simulink model "Thesis_model"  (R2023b)
settings: Solver=FixedStepAuto  StartTime=0  StopTime=24*3600*3  FixedStep=3600  RelTol=1e-3
undefined symbols (not defined in the file): C_Battery_kWh, Davies, demand, Hay, Max_charge_potential, P_Inv_W_max, path_carnot, phase, plugin_out, PV_W, req_charge, req_SOC
libraries: carnot x13, rllib x1
settings Model: Creator=Rohan  LastModifiedBy=Rohan
settings SolverCC: EnableFixedStepZeroCrossing=on

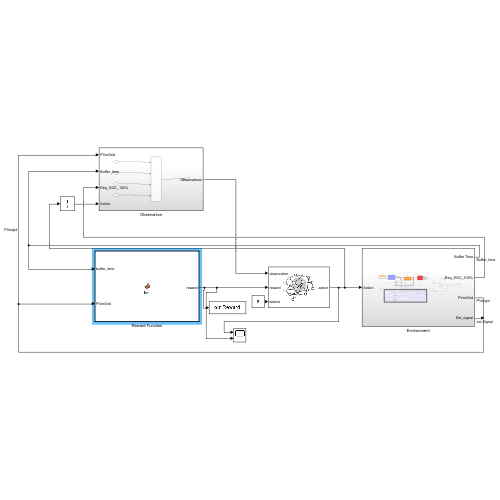
[thumbnail: Simulink's stored preview of the top-level diagram]
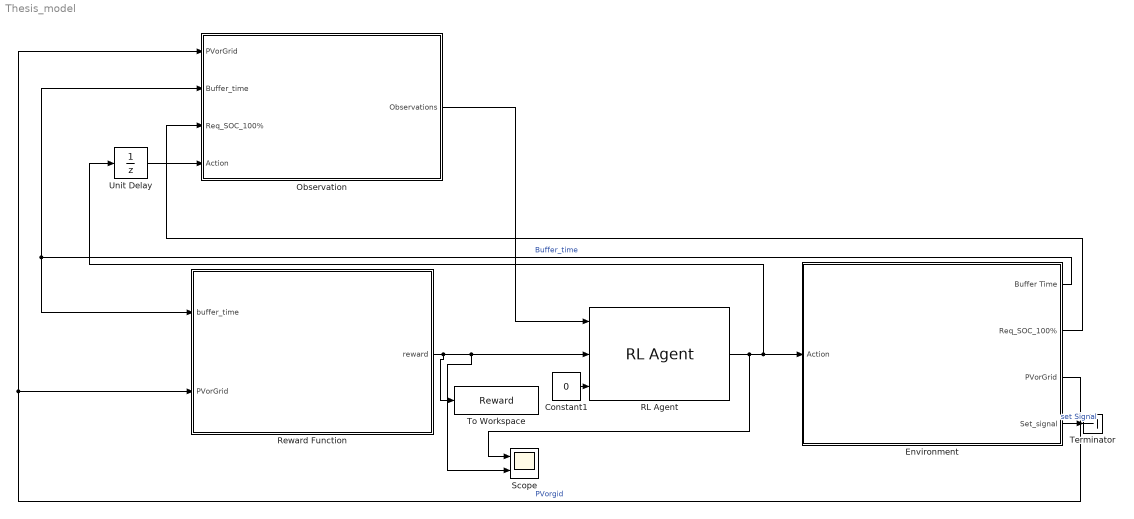
== system Thesis_model ==
  Constant1 : Constant  Value=0
  Environment : Subsystem
  Observation : Subsystem
  RL Agent : rllib/RL Agent  Agent=agentDQN_Trained  ExternalActionAsInput=off  ProvideLastAction=off  ProvideCumRwd=off  TreatAsDirectFeedthrough=on  UseStrictObservationDataTypes=off
  Reward Function : MATLAB Function  TreatAsAtomicUnit=on
  Scope : Scope  NumInputPorts=2
  Terminator : Terminator
  To Workspace : ToWorkspace  VariableName=Reward  SampleTime=-1
  Unit Delay : UnitDelay  SampleTime=-1  HasFrameUpgradeWarning=on
  wires:
  Reward Function/1(reward) -> To Workspace/1, Scope/2, RL Agent/2
  Environment/1(Buffer Time) -> Observation/2(Buffer_time), Reward Function/1(buffer_time)  "Buffer_time"
  Observation/1(Observations) -> RL Agent/1
  Constant1/1 -> RL Agent/3
  Environment/2(Req_SOC_100%) -> Observation/3(Req_SOC_100%)
  Environment/3(PVorGrid) -> Observation/1(PVorGrid), Reward Function/2(PVorGrid)  "PVorgid"
  RL Agent/1 -> Scope/1, Environment/1(Action), Unit Delay/1
  Unit Delay/1 -> Observation/4(Action)
  Environment/4(Set_signal) -> Terminator/1  "set Signal"

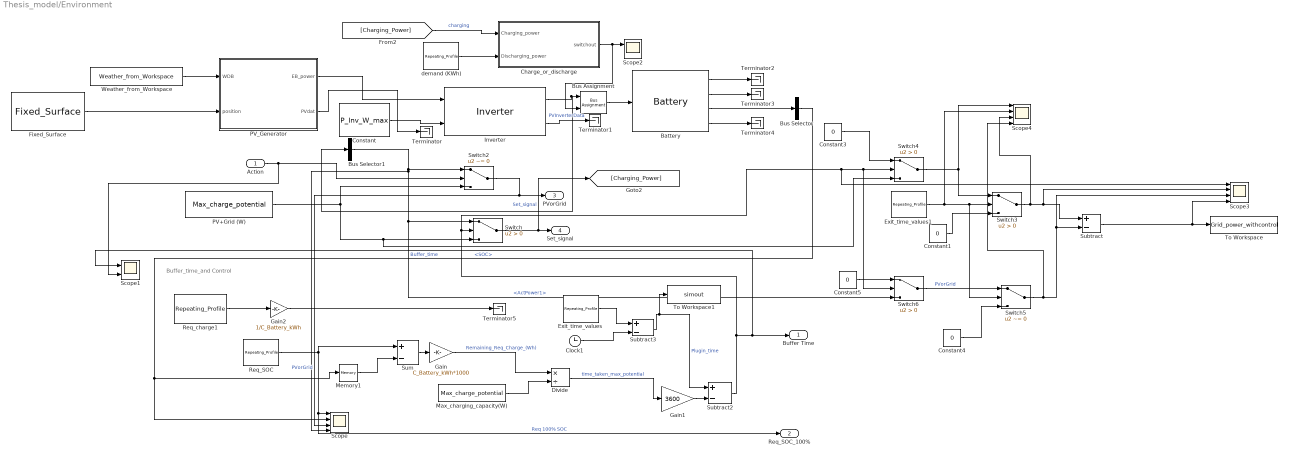
== system Thesis_model/Environment ==
  note: Buffer_time_and Control
  Action : Inport
  Battery : carnot/Storage/Electric/Battery  cap_kWh=C_Battery_kWh  eta_ch=1  eta_dis=1  cap0=Initial_SOC  SOC_max=1  SOC_min=0  Pmax=10000  Pmin=-10000  P_standby=0
      settings: SourceProductName=Carnot
  Bus Assignment : BusAssignment  AssignedSignals=ActPower1
  Bus Selector : BusSelector  OutputSignals=SOC
  Bus Selector1 : BusSelector  OutputSignals=ActPower1
  Charge_or_discharge : Subsystem
  Clock1 : Clock
  Constant : Constant  Value=P_Inv_W_max
  Constant{1,3..5} (4 alike) : Constant  Value=0
  Divide : Product  Inputs=*/
  Exit_time_values : carnot/Load/General/Repeating_Profile  period=plugin_out(end,1)  rep_seq_t=plugin_out(:,1)'  rep_seq_d=[1 ]*3600  rep_seq_y=plugin_out(:,2)'
      settings: SourceProductName=Carnot
  Exit_time_values1 : carnot/Load/General/Repeating_Profile  period=plugin_out(end,1)  rep_seq_t=plugin_out(:,1)'  rep_seq_d=[1 ]*3600  rep_seq_y=plugin_out(:,2)'
      settings: SourceProductName=Carnot
  Fixed_Surface : carnot/Weather/Fixed_Surface  colangle=30  colazi=0  colrot=0
      settings: SourceProductName=Carnot
  Gain : Gain  Gain=C_Battery_kWh*1000
  Gain1 : Gain  Gain=3600
  Gain2 : Gain  Gain=1/C_Battery_kWh
  Inverter : carnot/Source/Electric_Generator/Inverter  PathName=fullfile(path_carnot('libsl'), 'Source','Electric_Generator','Inverter','parameter_set')  FileName='<user defined>'  userPath=off  userParam=on  Pacnom=P_Inv_W  nphase=1-phase  U=230  f=50  PstepsEta=[0 0.1 0.2 0.25 0.3 0.5 0.75 1]  Eta=[0 0.948 0.966 0.969 0.97 0.972 0.97 0.967]  P_standby=0
      settings: SourceProductName=Carnot
  Max_charging_capacity(W) : Constant  Value=Max_charge_potential
  Memory1 : Memory
  PV+Grid (W) : Constant  Value=Max_charge_potential
  PV_Generator : Subsystem  AncestorBlock=carnot/Source/Electric_Generator/PV_Generator  mask(PV_Module_simple){Wp=PV_W, delta_Wp_K=0.0047, fgen=0.91 % 0.06 power missmatch, 0.01 diodes, 0.02 data sheet tolerance}
      mask prompts: Wp "Peak power of the generator [W]"; delta_Wp_K "Temperature coefficient Pmax 1/K"; fgen "efficiency generator field (lossses in diodes, power missmatch, dirt)"
      mask help:
      | This block simultes a PV module or generatater and calculates the DC power based on the parameters:
      | - Wp of one module or generator at STC [W]
      | - temperature coefficient of Pmax [1/K]
      | - dirt and degradation effects
      | The output DC power of the PV generator is ActPower1 in EB (power only)
      mask Help: web(fullfile(path_carnot('help'),'PV_Generator.html'),'-helpbrowser')
      mask Display: plot(0,0,100,100,[10,40,90,60,10],[10,90,90,10,10],[37,53,60,43,37],[70,70,86,86,70],[60,75,82,67,60],[70,71,86,86,70],[35,30,43,51,35],[65,50,49,65,65],[51,67,73,58,51],[50,50,66,66,50],[28,20,36,43,28],[41,23,23,41,41],[49,44,58,65,49],[41,23,22,41,41])
  Req_SOC : carnot/Load/General/Repeating_Profile  period=req_SOC(end,1)  rep_seq_t=req_SOC(:,1)'  rep_seq_d=[1 ]*3600  rep_seq_y=req_SOC(:,2)'
      settings: SourceProductName=Carnot
  Req_charge1 : carnot/Load/General/Repeating_Profile  period=req_charge(end,1)  rep_seq_t=req_charge(:,1)'  rep_seq_d=3600  rep_seq_y=req_charge(:,2)'
      settings: SourceProductName=Carnot
  Scope : Scope  NumInputPorts=4
  Scope1 : Scope  NumInputPorts=2
  Scope2 : Scope  NumInputPorts=2
  Scope3 : Scope  NumInputPorts=4
  Scope4 : Scope  NumInputPorts=4
  Subtract : Sum  Inputs=+-
  Subtract2 : Sum  Inputs=+-
  Subtract3 : Sum  Inputs=+-
  Sum : Sum  Inputs=|+-
  Switch : Switch  Criteria=u2 > Threshold  RndMeth=Zero  SaturateOnIntegerOverflow=off  InputSameDT=off
  Switch2 : Switch  Criteria=u2 ~= 0  Threshold=0.5  ZeroCross=off  SaturateOnIntegerOverflow=off  InputSameDT=off
  Switch3 : Switch  Criteria=u2 > Threshold  SaturateOnIntegerOverflow=off  InputSameDT=off
  Switch4 : Switch  Criteria=u2 > Threshold  ZeroCross=off  SaturateOnIntegerOverflow=off  InputSameDT=off
  Switch5 : Switch  Criteria=u2 ~= 0  SaturateOnIntegerOverflow=off  InputSameDT=off
  Switch6 : Switch  Criteria=u2 > Threshold  ZeroCross=off  SaturateOnIntegerOverflow=off  InputSameDT=off
  Terminator{,1..5} (6 alike) : Terminator
  To Workspace : ToWorkspace  VariableName=Grid_power_withcontrol  SampleTime=-1
  To Workspace1 : ToWorkspace  VariableName=simout  SaveFormat=Timeseries  SampleTime=-1
  Weather_from_Workspace : carnot/Weather/Weather_from_Workspace  file=weather
      settings: SourceProductName=Carnot
  demand (KWh) : carnot/Load/General/Repeating_Profile  period=demand(end,1)  rep_seq_t=demand(:,1)'  rep_seq_d=[1 ]*3600  rep_seq_y=demand(:,2)'
      settings: SourceProductName=Carnot
  Buffer Time : Outport
  Req_SOC_100% : Outport  Port=2
  PVorGrid : Outport  Port=3
  Set_signal : Outport  Port=4
  wires:
  PV_Generator/1(EB_power) -> Inverter/1
  PV_Generator/2(PVdat) -> Terminator/1
  Fixed_Surface/1 -> PV_Generator/2(position)
  Inverter/2 -> Terminator1/1  "PVInverterData"
  Constant/1 -> Inverter/2
  Bus Selector1/1 -> Switch6/3, Switch/1, Scope/4, Switch2/1  "<ActPower1>"
  Weather_from_Workspace/1 -> PV_Generator/1(WDB)
  Charge_or_discharge/1(switchout) -> Bus Assignment/2, Scope2/1
  [Charging_Power] -> Charge_or_discharge/1(Charging_power)  "charging"
  Bus Assignment/1 -> Battery/1
  demand (KWh)/1 -> Charge_or_discharge/2(Discharging_power)
  PV+Grid (W)/1 -> Switch4/3, Switch/3, Switch2/3
  Switch2/1 -> PVorGrid/1, Scope/3  "PVorGrid"
  Action/1 -> Scope1/2, Switch2/2
  Battery/3 -> Bus Selector/1
  Bus Selector/1 -> Memory1/1, Scope/2  "<SOC>"
  Battery/1 -> Terminator2/1
  Battery/2 -> Terminator3/1
  Battery/4 -> Terminator4/1
  Exit_time_values/1 -> Subtract3/1
  Switch/1 -> [Charging_Power], Set_signal/1  "Set_signal"
  Inverter/1 -> Bus Assignment/1, Bus Selector1/1
  Req_SOC/1 -> Req_SOC_100%/1, Scope/1, Sum/1  "Req 100% SOC"
  Subtract2/1 -> Scope3/1, Switch6/2, Switch4/2, Switch/2, Scope1/1, Buffer Time/1  "Buffer_time"
  Sum/1 -> Gain/1
  Gain2/1 -> Terminator5/1
  Subtract3/1 -> To Workspace1/1, Subtract2/1  "Plugin_time"
  Gain1/1 -> Subtract2/2
  Gain/1 -> Divide/1  "Remaining_Req_Charge_(Wh)"
  Max_charging_capacity(W)/1 -> Divide/2
  Req_charge1/1 -> Gain2/1
  Divide/1 -> Gain1/1  "time_taken_max_potential"
  Clock1/1 -> Subtract3/2
  Memory1/1 -> Sum/2
  Subtract/1 -> Scope3/4, To Workspace/1
  Switch3/1 -> Scope4/3, Scope3/2, Subtract/1
  Constant1/1 -> Switch3/3
  Constant3/1 -> Switch4/1
  Switch4/1 -> Switch3/1, Scope4/1
  Constant4/1 -> Switch5/3
  Constant5/1 -> Switch6/1
  Switch6/1 -> Switch5/1  "PVorGrid"
  Switch5/1 -> Scope4/4, Scope3/3, Subtract/2
  Exit_time_values1/1 -> Scope4/2, Switch5/2, Switch3/2

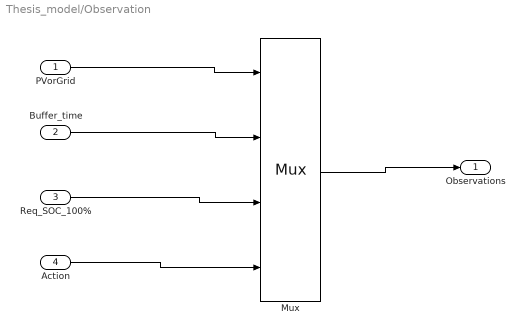
== system Thesis_model/Observation ==
  PVorGrid : Inport
  Buffer_time : Inport  Port=2
  Req_SOC_100% : Inport  Port=3
  Action : Inport  Port=4
  Mux : Mux
  Observations : Outport
  wires:
  Req_SOC_100%/1 -> Mux/3
  Buffer_time/1 -> Mux/2
  PVorGrid/1 -> Mux/1
  Mux/1 -> Observations/1
  Action/1 -> Mux/4

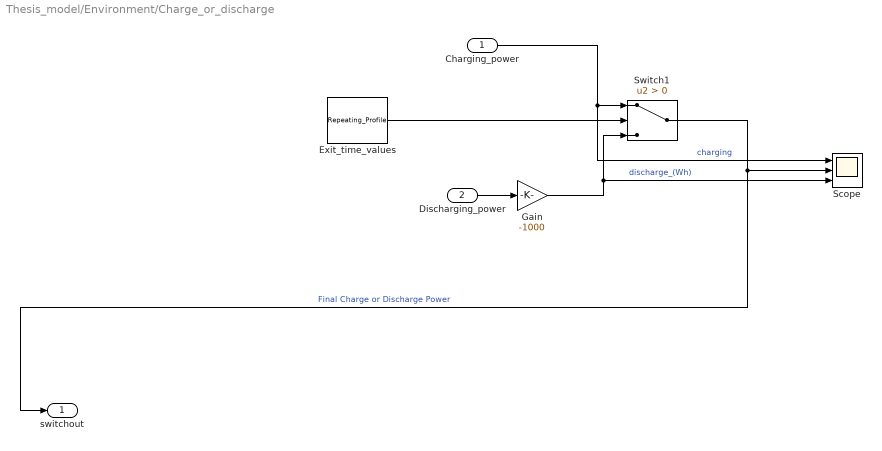
== system Thesis_model/Environment/Charge_or_discharge ==
  Charging_power : Inport
  Discharging_power : Inport  Port=2
  Exit_time_values : carnot/Load/General/Repeating_Profile  period=plugin_out(end,1)  rep_seq_t=plugin_out(:,1)'  rep_seq_d=[1 ]*3600  rep_seq_y=plugin_out(:,2)'
      settings: SourceProductName=Carnot
  Gain : Gain  Gain=-1000
  Scope : Scope  NumInputPorts=3
  Switch1 : Switch  Criteria=u2 > Threshold  SaturateOnIntegerOverflow=off  InputSameDT=off  OutDataTypeStr=Inherit: Same as first input
  switchout : Outport
  wires:
  Switch1/1 -> switchout/1, Scope/2  "Final Charge or Discharge Power"
  Charging_power/1 -> Scope/1, Switch1/1  "charging"
  Exit_time_values/1 -> Switch1/2
  Gain/1 -> Switch1/3, Scope/3  "discharge_(Wh)"
  Discharging_power/1 -> Gain/1

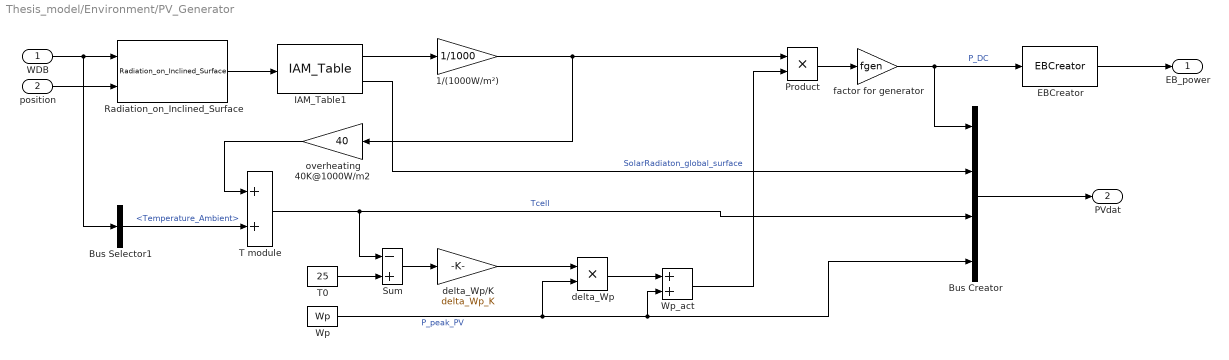
== system Thesis_model/Environment/PV_Generator ==
  WDB : Inport
  position : Inport  Port=2
  1/(1000W/m²) : Gain  Gain=1/1000
  Bus Creator : BusCreator  Inputs=4
  Bus Selector1 : BusSelector  OutputSignals=Temperature_Ambient
  EBCreator : carnot/Basic/Electric/EBCreator  Inport_ID=off  Inport_f=off  Inport_v1=off  Inport_p1=on  Inport_pf1=off  Inport_v2=off  Inport_p2=off  Inport_pf2=off  Inport_v3=off  Inport_p3=off  Inport_pf3=off  ID=1  f=0  v1=0  p1=1e5  pf1=1  v2=0  p2=0  pf2=0  v3=0  p3=0  pf3=0  Annotation_ID=off  Annotation_f=off  Annotation_v1=off  Annotation_p1=off  Annotation_pf1=off  Annotation_v2=off  Annotation_p2=off  Annotation_pf2=off  Annotation_v3=off  Annotation_p3=off  Annotation_pf3=off
      settings: SourceProductName=Carnot
  IAM_Table1 : carnot/Source/Solar_Thermal/IncidenceAngleModifier/IAM_Table  fta=1  angle=[0:5:90]  Kb="[1.0000    1.0000    0.9999    0.9996    0.9991    0.9982    0.9965  0.9935    0.9886    0.9807    0.9678    0.9473    0.9148    0.8638   0.7846    0.6644    0.4907    0.2599    0.0000]"  Kd=0.915
      settings: SourceProductName=Carnot
  Product : Product  RndMeth=Zero
  Radiation_on_Inclined_Surface : carnot/Weather/Radiation_on_Inclined_Surface  sky=Hay-Davies  reflect=0.2
      settings: SourceProductName=Carnot
  Sum : Sum  Inputs=-+
  T module : Sum  Inputs=2
  T0 : Constant  Value=25
  Wp : Constant  Value=Wp
  Wp_act : Sum
  delta_Wp : Product  RndMeth=Zero
  delta_Wp/K : Gain  Gain=delta_Wp_K
  factor for generator : Gain  Gain=fgen
  overheating 40K@1000W/m2 : Gain  Gain=40
  EB_power : Outport  VectorParamsAs1DForOutWhenUnconnected=off
  PVdat : Outport  Port=2  VectorParamsAs1DForOutWhenUnconnected=off
  wires:
  IAM_Table1/2 -> Bus Creator/2  "SolarRadiaton_global_surface"
  position/1 -> Radiation_on_Inclined_Surface/2
  Radiation_on_Inclined_Surface/1 -> IAM_Table1/1
  WDB/1 -> Radiation_on_Inclined_Surface/1, Bus Selector1/1
  factor for generator/1 -> EBCreator/1, Bus Creator/1  "P_DC"
  delta_Wp/K/1 -> delta_Wp/1
  Product/1 -> factor for generator/1
  1/(1000W/m²)/1 -> Product/1, overheating 40K@1000W/m2/1
  Wp_act/1 -> Product/2
  T module/1 -> Sum/1, Bus Creator/3  "Tcell"
  IAM_Table1/1 -> 1/(1000W/m²)/1
  T0/1 -> Sum/2
  Sum/1 -> delta_Wp/K/1
  overheating 40K@1000W/m2/1 -> T module/1
  Bus Selector1/1 -> T module/2  "<Temperature_Ambient>"
  Wp/1 -> Wp_act/2, Bus Creator/4, delta_Wp/2  "P_peak_PV"
  delta_Wp/1 -> Wp_act/1
  Bus Creator/1 -> PVdat/1
  EBCreator/1 -> EB_power/1

== matlab function Thesis_model/Reward Function ==
  data: buffer_time input; reward output; PVorGrid input
function reward = fcn(buffer_time,PVorGrid)
reward=0;     
     if buffer_time<=0 && PVorGrid==8000
        reward=1;  %Grid is good
     elseif buffer_time>0 && PVorGrid~=8000
       reward=1 ;  %PV is good
     elseif buffer_time<=0 && PVorGrid~=8000
    reward=-2;% PV is Bad
     else
         reward=-2; %Grid is bad
     end
% % 
% % % For Minimum Chargining/Emergency case condition %
% % 
% %     if current_SOC<Emergency_charge && Action>=0.5 %PV
% %         reward2=-2;
% %     elseif current_SOC<Emergency_charge && Action<0.5 %Grid+PV
% %         reward2=1;
% %     end
 % else %Car Disconnected (Discharging)
 %     reward=reward+0;
